simulink model "gm_wahWahEffect"  (R2022b)
settings: Solver=FixedStepDiscrete  StartTime=0.0  StopTime=simParams.stopTime  RelTol=1e-3
PostLoadFcn:
  | postLoadCallback
InitFcn:
  | initCallback
StopFcn:
  | stopCallback
undefined symbols (not defined in the file or in its folder): modelParams
libraries: dspsigops x11, dspsrcs4 x8, hdlmdlgenlib x2
(part 2 of 2)

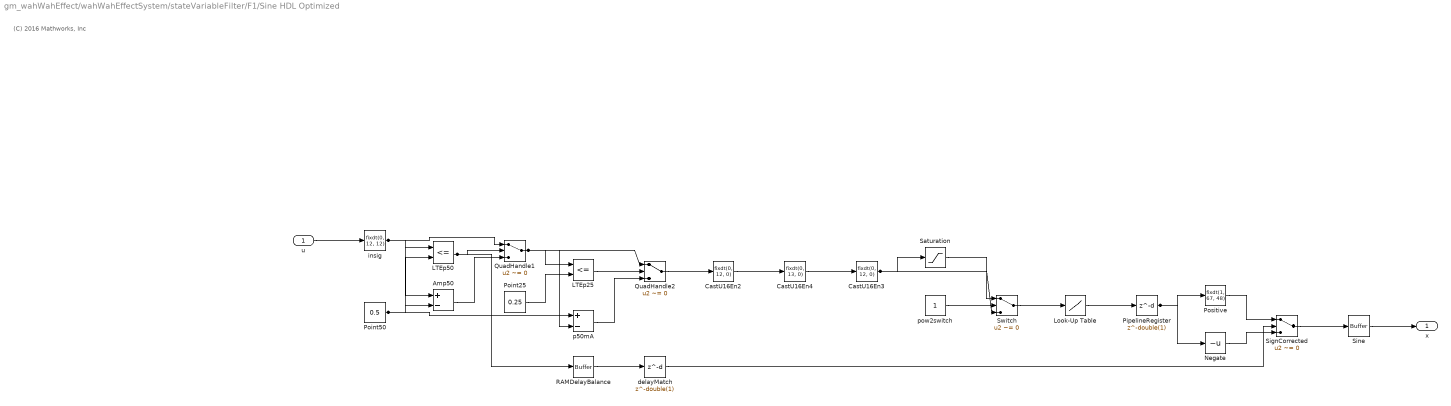
== system gm_wahWahEffect/wahWahEffectSystem/stateVariableFilter/F1/Sine HDL Optimized ==
  note: (C) 2016 Mathworks, Inc
  u : Inport  OutDataTypeStr=fixdt(1, 66, 48)  SampleTime=1.01725260416667e-08
  Amp50 : Sum  Inputs=+-  AccumDataTypeStr=fixdt(1, 68, 67)  OutDataTypeStr=fixdt(1, 68, 67)  SampleTime=1.01725260416667e-08
  CastU16En2 : DataTypeConversion  OutDataTypeStr=fixdt(0, 12, 0)  ConvertRealWorld=Stored Integer (SI)  SampleTime=1.01725260416667e-08  SaturateOnIntegerOverflow=off  RndMeth=Floor
  CastU16En3 : DataTypeConversion  OutDataTypeStr=fixdt(0, 12, 0)  ConvertRealWorld=Stored Integer (SI)  SampleTime=1.01725260416667e-08  RndMeth=Floor
  CastU16En4 : DataTypeConversion  OutDataTypeStr=fixdt(0, 13, 0)  SampleTime=1.01725260416667e-08  SaturateOnIntegerOverflow=off  RndMeth=Floor
  LTEp25 : RelationalOperator  Operator=<=  OutDataTypeStr=boolean  SampleTime=1.01725260416667e-08  InputSameDT=off
  LTEp50 : RelationalOperator  Operator=<=  OutDataTypeStr=boolean  SampleTime=1.01725260416667e-08  InputSameDT=off
  Look-Up Table : Lookup_n-D  NumberOfTableDimensions=1  BreakpointsForDimension1="fi(\"numerictype\",numerictype(0,12,0),\"fimath\",fimath(\"RoundingMethod\", \"Floor\",\"OverflowAction\", \"Wrap\",\"ProductMode\",\"FullPrecision\",\"SumMode\",\"FullPrecision\"),\"Value\",\"[0 1 2 3 4 5 6 7 8 9 10 11 12 13 14 15 16 17 18 19 20 21 22 23 24 25 26 27 28 29 30 31 32 33 34 35 36 37 38 39 40 41 42 43 44 45 46 47 48 49 50 51 52 53 54 55 56 57 58 59 60 61 62 63 64 65 66 67 68 69 70 71 72 73 74 75 76 77 78 79 80 81 82 83 84 85 86 87 88 89 90 91 92 93 94 95 96 97 98 99 100 101 102 103 104 105 106 107 108 109 110 111 112 113 114 115 116 117 118 119 120 121 122 123 124 125 126 127 128 129 130 131 132 133 134 135 136 137 138 139 140 141 142 143 144 145 146 147 148 149 150 151 152 153 154 155 156 157 158 159 160 161 162 163 164 165 166 167 168 169 170 171 172 173 174 175 176 177 178 179 180 181 182 183 184 185 186 187 188 189 190 191 192 193 194 195 196 197 198 199 200 201 202 203 204 205 206 207 208 209 210 211 212 213 214 215 216 217 218 219 220 221 222 223 224 225 226 227 228 229 230 231 232 233 234 235 236 237 238 239 240 241 242 243 244 245 246 247 248 249 250 251 252 253 254 255 256 257 258 259 260 261 262 263 264 265 266 267 268 269 270 271 272 273 274 275 276 277 278 279 280 281 282 283 284 285 286 287 288 289 290 291 292 293 294 295 296 297 298 299 300 301 302 303 304 305 306 307 308 309 310 311 312 313 314 315 316 317 318 319 320 321 322 323 324 325 326 327 328 329 330 331 332 333 334 335 336 337 338 339 340 341 342 343 344 345 346 347 348 349 350 351 352 353 354 355 356 357 358 359 360 361 362 363 364 365 366 367 368 369 370 371 372 373 374 375 376 377 378 379 380 381 382 383 384 385 386 387 388 389 390 391 392 393 394 395 396 397 398 399 400 401 402 403 404 405 406 407 408 409 410 411 412 413 414 415 416 417 418 419 420 421 422 423 424 425 426 427 428 429 430 431 432 433 434 435 436 437 438 439 440 441 442 443 444 445 446 447 448 449 450 451 452 453 454 455 456 457 458 459 460 461 462 463 464 465 466 467 468 469 470 471 472 473 474 475 476 477 478 479 480 481 482 483 484 485 486 487 488 489 490 491 492 493 494 495 496 497 498 499 500 501 502 503 504 505 506 507 508 509 510 511 512 513 514 515 516 517 518 519 520 521 522 523 524 525 526 527 528 529 530 531 532 533 534 535 536 537 538 539 540 541 542 543 544 545 546 547 548 549 550 551 552 553 554 555 556 557 558 559 560 561 562 563 564 565 566 567 568 569 570 571 572 573 574 575 576 577 578 579 580 581 582 583 584 585 586 587 588 589 590 591 592 593 594 595 596 597 598 599 600 601 602 603 604 605 606 607 608 609 610 611 612 613 614 615 616 617 618 619 620 621 622 623 624 625 626 627 628 629 630 631 632 633 634 635 636 637 638 639 640 641 642 643 644 645 646 647 648 649 650 651 652 653 654 655 656 657 658 659 660 661 662 663 664 665 666 667 668 669 670 671 672 673 674 675 676 677 678 679 680 681 682 683 684 685 686 687 688 689 690 691 692 693 694 695 696 697 698 699 700 701 702 703 704 705 706 707 708 709 710 711 712 713 714 715 716 717 718 719 720 721 722 723 724 725 726 727 728 729 730 731 732 733 734 735 736 737 738 739 740 741 742 743 744 745 746 747 748 749 750 751 752 753 754 755 756 757 758 759 760 761 762 763 764 765 766 767 768 769 770 771 772 773 774 775 776 777 778 779 780 781 782 783 784 785 786 787 788 789 790 791 792 793 794 795 796 797 798 799 800 801 802 803 804 805 806 807 808 809 810 811 812 813 814 815 816 817 818 819 820 821 822 823 824 825 826 827 828 829 830 831 832 833 834 835 836 837 838 839 840 841 842 843 844 845 846 847 848 849 850 851 852 853 854 855 856 857 858 859 860 861 862 863 864 865 866 867 868 869 870 871 872 873 874 875 876 877 878 879 880 881 882 883 884 885 886 887 888 889 890 891 892 893 894 895 896 897 898 899 900 901 902 903 904 905 906 907 908 909 910 911 912 913 914 915 916 917 918 919 920 921 922 923 924 925 926 927 928 929 930 931 932 933 934 935 936 937 938 939 940 941 942 943 944 945 946 947 948 949 950 951 952 953 954 955 956 957 958 959 960 961 962 963 964 965 966 967 968 969 970 971 972 973 974 975 976 977 978 979 980 981 982 983 984 985 986 987 988 989 990 991 992 993 994 995 996 997 998 999 1000 1001 1002 1003 1004 1005 1006 1007 1008 1009 1010 1011 1012 1013 1014 1015 1016 1017 1018 1019 1020 1021 1022 1023]\")"  Table="reshape(fi(\"numerictype\",numerictype(1,67,48),\"fimath\",fimath(\"RoundingMethod\", \"Floor\",\"OverflowAction\", \"Wrap\",\"ProductMode\",\"FullPrecision\",\"SumMode\",\"FullPrecision\"),\"Value\",\"[0;0.001533980186284367164262;0.003067956762965451389391;0.004601926120447075163611;0.006135884649154377257219;0.007669828739530260008905;0.009203754782060258321508;0.01073765916726543423465;0.01227153828572014049314;0.01380538852805912597432;0.01533920628498819382912;0.01687298794728064876836;0.01840672990580571877217;0.01994042855151434423533;0.02147408027547115239031;0.0230076814688402464526;0.02454122852291362733013;0.02607471782910408819589;0.02760814577896653077005;0.02914150876419441260623;0.03067480317663751065993;0.03220802540830547400219;0.03374117185137848196064;0.03527423889821434954683;0.03680722294135918559732;0.0383401203735509454873;0.03987292758774074741268;0.04140564097707510882174;0.04293825693494213169288;0.04447077185493952811157;0.0460031821309137001208;0.04753548415695973972106;0.04906767432741787615669;0.05059974903689834491161;0.05213170468028494042301;0.05366353765273146336767;0.0551952443496901423714;0.05672682116690808129533;0.05825826450043436466331;0.05978957074664137394393;0.06132073630220702398219;0.06285175756416094827728;0.06438263092985607727314;0.06591335279700416549531;0.06744391956366513340981;0.06897432762826838370529;0.07050457338961280129297;0.07203465324688806958875;0.07356456359966756508584;0.07509430084792256820947;0.07662386139203292145794;0.07815324163279413482996;0.07968243797143159667939;0.08121144680959346828786;0.08274026454937555286051;0.08426888759332484823972;0.08579731234443954690505;0.08732553520619035225536;0.08885355258252403132246;0.09038136087786341477113;0.09190895649713226589483;0.09343633584574817518842;0.09496349532964032391646;0.09649043135525303682698;0.09801714032955999300611;0.09954361866006777859184;0.101069862754826544915;0.1025958690224371139266;0.1041216338720545309116;0.1056471537134093807708;0.1071724249568077880213;0.108697444013138522223;0.1102222072938836561207;0.1117467112111256710705;0.1132709521775652206088;0.1147949266065104723111;0.1163186309119055295014;0.1178420615083233258247;0.119365214810990494243;0.1208880872357767088943;0.1224106751992160013742;0.123932975118513866164;0.12545498341154726063;0.1269766964968859213059;0.1284981107937923638929;0.1300192227222325414004;0.1315400287028829495739;0.1330605251571377323216;0.1345807085071264452836;0.1361005751757069504038;0.1376201215864867322125;0.13913934416382645054;0.1406582393328505986574;0.1421768035194475032768;0.1436950331502941935469;0.1452129246528457429122;0.1467304744553601381085;0.1482476789868947264495;0.149764534677320426681;0.1512810379573288344091;0.1527971852584428802402;0.1543129730130203824956;0.155828397654264705352;0.1573434556162389696965;0.1588581433338625004126;0.1603724572429285899489;0.1618863937801116037463;0.1633999493829740856654;0.1649131204899703107003;0.1664259035404640485467;0.1679382949747321163159;0.1694502912339679312481;0.170961888760302826995;0.1724730839967953954783;0.173983873387463461313;0.1754942533772698709527;0.1770042204121473616851;0.1785137709389985616326;0.1800229014056995424653;0.1815316082611246883971;0.1830398879551395907583;0.1845477369386188115641;0.1860551516634458835142;0.1875621285825310735618;0.1890686641498078301993;0.1905747548202540997409;0.1920803970498923263222;0.1935855872958036627551;0.195090322016127970528;0.1965945976700815833738;0.1980984107179537545562;0.1996017576211315258661;0.2011046348420926221934;0.2026070388444196623823;0.2041089660928179227994;0.2056104130530975737656;0.2071113761922198648335;0.2086118519782651503647;0.2101118368804684166662;0.2116113273692263874182;0.2131103199160904182463;0.214608810993787813004;0.2161067970762182710587;0.2176042746384823090011;0.2191012401568706025046;0.2205976901088746444657;0.222093620973204508573;0.2235890292297888493067;0.2250839113597926655075;0.2265782638456101949487;0.2280720831708862306186;0.2295653658205196734343;0.2310581082806706376687;0.2325503070387746618053;0.2340419585835427085385;0.2355330594049753756281;0.2370236059943664486127;0.2385135948443171116651 ...(+21554 chars)]\"), [1  1024])"  InterpMethod=Flat  ExtrapMethod=Clip  DiagnosticForOutOfRangeInput=Error  SampleTime=1.01725260416667e-08  OutDataTypeStr=fixdt(1, 67, 48)
  Negate : UnaryMinus  SampleTime=1.01725260416667e-08
  PipelineRegister : Delay  DelayLength=double(1)  InitialCondition=0  SampleTime=1.01725260416667e-08
  Point25 : Constant  Value=0.25  OutDataTypeStr=fixdt(0, 67, 67)  SampleTime=1.01725260416667e-08
  Point50 : Constant  Value=0.5  OutDataTypeStr=fixdt(0, 67, 67)  SampleTime=1.01725260416667e-08
  Positive : DataTypeConversion  OutDataTypeStr=fixdt(1, 67, 48)  SampleTime=1.01725260416667e-08  SaturateOnIntegerOverflow=off  RndMeth=Floor
  QuadHandle1 : Switch  Criteria=u2 ~= 0  Threshold=double(0)  OutDataTypeStr=fixdt(1, 68, 67)  SampleTime=1.01725260416667e-08  SaturateOnIntegerOverflow=off  InputSameDT=off
  QuadHandle2 : Switch  Criteria=u2 ~= 0  Threshold=double(0)  OutDataTypeStr=fixdt(0, 12, 12)  SampleTime=1.01725260416667e-08  SaturateOnIntegerOverflow=off  InputSameDT=off
  RAMDelayBalance : hdlmdlgenlib/Buffer
  Saturation : Saturate  UpperLimit="fi(0,0,12,0,\"hex\",\"3ff\")"  LowerLimit="fi(0,0,12,0,\"hex\",\"000\")"  SampleTime=1.01725260416667e-08  OutDataTypeStr=fixdt(0, 12, 0)
  SignCorrected : Switch  Criteria=u2 ~= 0  Threshold=double(0)  OutDataTypeStr=fixdt(1, 67, 48)  SampleTime=1.01725260416667e-08  SaturateOnIntegerOverflow=off  InputSameDT=off
  Sine : hdlmdlgenlib/Buffer
  Switch : Switch  Criteria=u2 ~= 0  Threshold=double(0)  OutDataTypeStr=fixdt(0, 12, 0)  SampleTime=1.01725260416667e-08  SaturateOnIntegerOverflow=off  InputSameDT=off
  delayMatch : Delay  DelayLength=double(1)  InitialCondition=0  SampleTime=1.01725260416667e-08
  insig : DataTypeConversion  OutDataTypeStr=fixdt(0, 12, 12)  SampleTime=1.01725260416667e-08  SaturateOnIntegerOverflow=off  RndMeth=Floor
  p50mA : Sum  Inputs=+-  AccumDataTypeStr=fixdt(1, 69, 67)  OutDataTypeStr=fixdt(1, 69, 67)  SampleTime=1.01725260416667e-08
  pow2switch : Constant  OutDataTypeStr=boolean  SampleTime=1.01725260416667e-08
  x : Outport  SampleTime=1.01725260416667e-08
  wires:
  Sine/1 -> x/1
  Amp50/1 -> QuadHandle1/3
  CastU16En2/1 -> CastU16En4/1
  CastU16En3/1 -> Switch/3, Saturation/1
  CastU16En4/1 -> CastU16En3/1
  LTEp25/1 -> QuadHandle2/2
  LTEp50/1 -> QuadHandle1/2, RAMDelayBalance/1
  PipelineRegister/1 -> Positive/1, Negate/1
  Negate/1 -> SignCorrected/3
  Point25/1 -> LTEp25/2
  Point50/1 -> p50mA/1, LTEp50/2, Amp50/2
  Positive/1 -> SignCorrected/1
  QuadHandle1/1 -> p50mA/2, QuadHandle2/1, LTEp25/1
  QuadHandle2/1 -> CastU16En2/1
  delayMatch/1 -> SignCorrected/2
  Saturation/1 -> Switch/1
  SignCorrected/1 -> Sine/1
  Switch/1 -> Look-Up Table/1
  insig/1 -> QuadHandle1/1, LTEp50/1, Amp50/1
  p50mA/1 -> QuadHandle2/3
  pow2switch/1 -> Switch/2
  RAMDelayBalance/1 -> delayMatch/1
  u/1 -> insig/1
  Look-Up Table/1 -> PipelineRegister/1
